simulink model "simulacionesProtesis"  (R2021a)
settings: Solver=VariableStepAuto  StartTime=0.0  StopTime=50  RelTol=1e-3
settings Model: Creator=jmata  LastModifiedBy=jmata

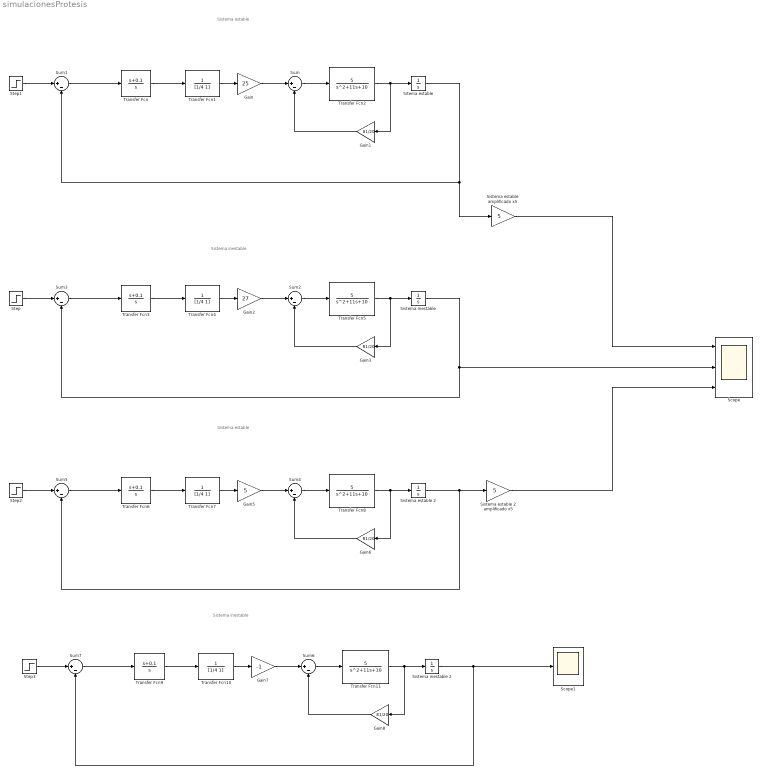
== system simulacionesProtesis ==
  note: Sistema inestable
  note: Sistema estable
  note: Sistema estable
  note: Sistema inestable
  Gain : Gain  Gain=25
  Gain{1,3,6,8} (4 alike) : Gain  Gain=81/20
  Gain2 : Gain  Gain=27
  Gain5 : Gain  Gain=5
  Gain7 : Gain  Gain=-1
  Scope : Scope  NumInputPorts=3
  Scope1 : Scope
  Sistema estable 2 : Integrator
  Sistema estable 2 amplificado x5 : Gain  Gain=5
  Sistema estable amplificado x5 : Gain  Gain=5
  Sistema inestable : Integrator
  Sistema inestable 2 : Integrator
  Sitema estable : Integrator
  Step : Step  Time=0  SampleTime=0
  Step1 : Step  Time=0  SampleTime=0
  Step2 : Step  SampleTime=0
  Step3 : Step  SampleTime=0
  Sum{,1..7} (8 alike) : Sum  Inputs=|+-
  Transfer Fcn{,3,6,9} (4 alike) : TransferFcn  Numerator=[1 0.1]  Denominator=[1 0]
  Transfer Fcn{1,4,7,10} (4 alike) : TransferFcn  Denominator=[1/4 1]
  Transfer Fcn{2,5,8,11} (4 alike) : TransferFcn  Numerator=[5]  Denominator=[1 11 10]
  wires:
  Sum1/1 -> Transfer Fcn/1
  Transfer Fcn/1 -> Transfer Fcn1/1
  Transfer Fcn1/1 -> Gain/1
  Gain/1 -> Sum/1
  Gain1/1 -> Sum/2
  Sum/1 -> Transfer Fcn2/1
  Transfer Fcn2/1 -> Gain1/1, Sitema estable/1
  Sitema estable/1 -> Sistema estable amplificado x5/1, Sum1/2
  Step1/1 -> Sum1/1
  Step/1 -> Sum3/1
  Sum2/1 -> Transfer Fcn5/1
  Gain3/1 -> Sum2/2
  Sistema inestable/1 -> Sum3/2, Scope/2
  Transfer Fcn5/1 -> Gain3/1, Sistema inestable/1
  Sum3/1 -> Transfer Fcn3/1
  Transfer Fcn3/1 -> Transfer Fcn4/1
  Transfer Fcn4/1 -> Gain2/1
  Gain2/1 -> Sum2/1
  Sistema estable amplificado x5/1 -> Scope/1
  Step2/1 -> Sum5/1
  Transfer Fcn8/1 -> Sistema estable 2/1, Gain6/1
  Sum4/1 -> Transfer Fcn8/1
  Gain6/1 -> Sum4/2
  Gain5/1 -> Sum4/1
  Transfer Fcn7/1 -> Gain5/1
  Transfer Fcn6/1 -> Transfer Fcn7/1
  Sum5/1 -> Transfer Fcn6/1
  Sum7/1 -> Transfer Fcn9/1
  Transfer Fcn9/1 -> Transfer Fcn10/1
  Transfer Fcn10/1 -> Gain7/1
  Gain7/1 -> Sum6/1
  Gain8/1 -> Sum6/2
  Sum6/1 -> Transfer Fcn11/1
  Transfer Fcn11/1 -> Gain8/1, Sistema inestable 2/1
  Step3/1 -> Sum7/1
  Sistema estable 2/1 -> Sistema estable 2 amplificado x5/1, Sum5/2
  Sistema estable 2 amplificado x5/1 -> Scope/3
  Sistema inestable 2/1 -> Sum7/2, Scope1/1
